simulink subsystem "local_waypoint_visualization"  (R2022b)
settings: Solver=VariableStepAuto  StartTime=0.0  StopTime=10.0  RelTol=1e-3
settings Model: Creator=USER  LastModifiedBy=USER

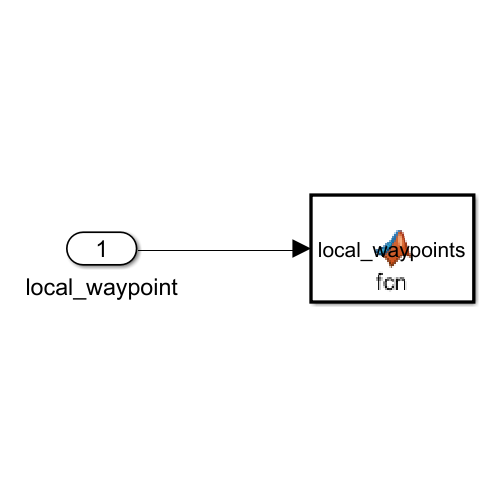
[thumbnail: Simulink's stored preview of the top-level diagram]
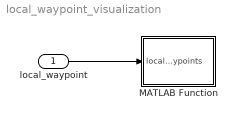
== system local_waypoint_visualization ==
  local_waypoint : Inport
  MATLAB Function : MATLAB Function  TreatAsAtomicUnit=on
  wires:
  local_waypoint/1 -> MATLAB Function/1(local_waypoints)

== matlab function local_waypoint_visualization/MATLAB Function ==
  data: local_waypoints input
function fcn(local_waypoints)
    filtered_matrix = local_waypoints(local_waypoints(:, 1) >= 0, :);
    filtered_matrix = filtered_matrix(filtered_matrix(:, 2) >= -20, :);
    filtered_matrix = filtered_matrix(filtered_matrix(:, 2) <= 20, :);
    
    scatter(filtered_matrix(:, 1), filtered_matrix(:, 2));
    xlim([-50, 50]);
    ylim([-50, 50]);

end
